simulink model "SolarLoRaWAN1"  (R2024b)
settings: Solver=VariableStepAuto  StartTime=0.0  StopTime=10.0  RelTol=1e-3
settings Model: Creator=ore.oluwatosin  LastModifiedBy=ore.oluwatosin

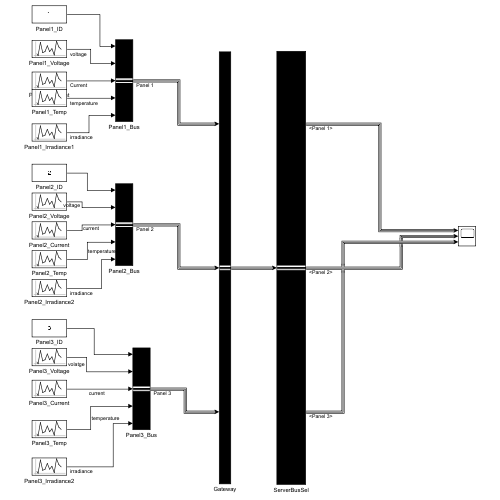
[thumbnail: Simulink's stored preview of the top-level diagram]
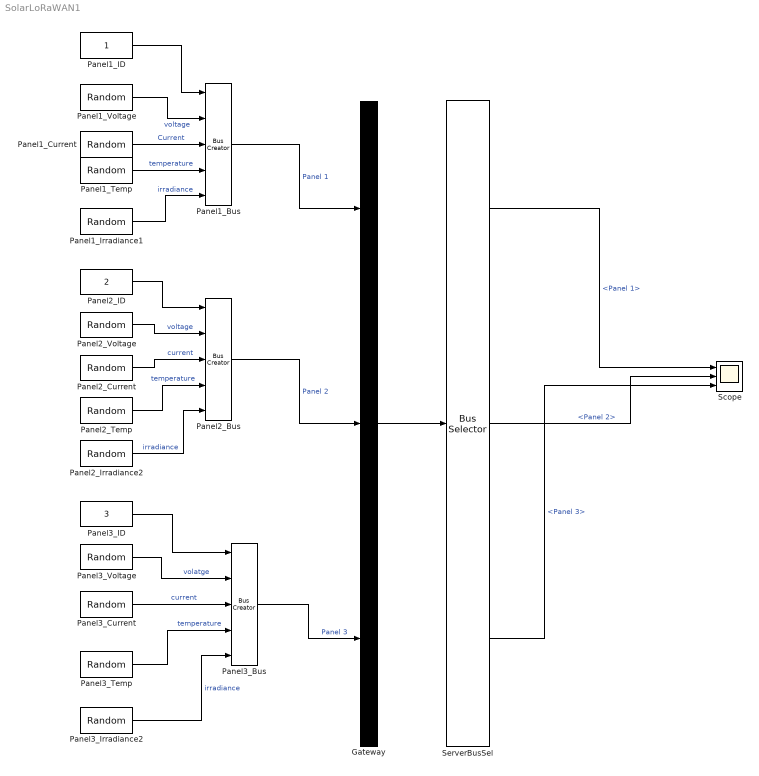
== system SolarLoRaWAN1 ==
  Gateway : BusCreator  Inputs=3
  Panel1_Bus : BusCreator  Inputs=5
  Panel1_Current : UniformRandomNumber  Minimum=8  Maximum=10  Seed=3  SampleTime=0.1
  Panel1_ID : Constant
  Panel1_Irradiance1 : UniformRandomNumber  Minimum=200  Maximum=1000  SampleTime=0.1
  Panel1_Temp : UniformRandomNumber  Minimum=25  Maximum=80  SampleTime=0.1
  Panel1_Voltage : UniformRandomNumber  Minimum=18  Maximum=36  SampleTime=0.1
  Panel2_Bus : BusCreator  Inputs=5
  Panel2_Current : UniformRandomNumber  Minimum=8  Maximum=10  Seed=10  SampleTime=0.1
  Panel2_ID : Constant  Value=2
  Panel2_Irradiance2 : UniformRandomNumber  Minimum=200  Maximum=1000  Seed=100  SampleTime=0.1
  Panel2_Temp : UniformRandomNumber  Minimum=25  Maximum=80  Seed=20  SampleTime=0.1
  Panel2_Voltage : UniformRandomNumber  Minimum=18  Maximum=36  Seed=10  SampleTime=0.1
  Panel3_Bus : BusCreator  Inputs=5
  Panel3_Current : UniformRandomNumber  Minimum=8  Maximum=10  SampleTime=0.1
  Panel3_ID : Constant  Value=3
  Panel3_Irradiance2 : UniformRandomNumber  Minimum=200  Maximum=1000  Seed=400  SampleTime=0.1
  Panel3_Temp : UniformRandomNumber  Minimum=25  Maximum=80  Seed=10  SampleTime=0.1
  Panel3_Voltage : UniformRandomNumber  Minimum=18  Maximum=36  Seed=5  SampleTime=0.1
  Scope : Scope  NumInputPorts=3
  ServerBusSel : BusSelector  OutputSignals=Panel 1,Panel 2,Panel 3
  wires:
  Panel1_ID/1 -> Panel1_Bus/1
  Panel1_Voltage/1 -> Panel1_Bus/2  "voltage"
  Panel1_Current/1 -> Panel1_Bus/3  "Current"
  Panel1_Temp/1 -> Panel1_Bus/4  "temperature"
  Panel2_ID/1 -> Panel2_Bus/1
  Panel2_Voltage/1 -> Panel2_Bus/2  "voltage"
  Panel2_Current/1 -> Panel2_Bus/3  "current"
  Panel2_Temp/1 -> Panel2_Bus/4  "temperature"
  Panel3_ID/1 -> Panel3_Bus/1
  Panel3_Voltage/1 -> Panel3_Bus/2  "volatge"
  Panel3_Current/1 -> Panel3_Bus/3  "current"
  Panel3_Temp/1 -> Panel3_Bus/4  "temperature"
  Panel1_Bus/1 -> Gateway/1  "Panel 1"
  Panel2_Bus/1 -> Gateway/2  "Panel 2"
  Panel3_Bus/1 -> Gateway/3  "Panel 3"
  Gateway/1 -> ServerBusSel/1
  ServerBusSel/1 -> Scope/1  "<Panel 1>"
  ServerBusSel/2 -> Scope/2  "<Panel 2>"
  ServerBusSel/3 -> Scope/3  "<Panel 3>"
  Panel1_Irradiance1/1 -> Panel1_Bus/5  "irradiance"
  Panel2_Irradiance2/1 -> Panel2_Bus/5  "irradiance"
  Panel3_Irradiance2/1 -> Panel3_Bus/5  "irradiance"
